simulink library "Plane_Movement_walk_right"  (R2024a)
settings: Solver=VariableStepAuto  StartTime=0.0  StopTime=10.0  RelTol=1e-3
undefined symbols (not defined in the file): Lower_limbs, Upper_limbs
libraries: functionAnglesSide x2, functionBezier_forward x1
settings Model: Creator=renre  LastModifiedBy=renre

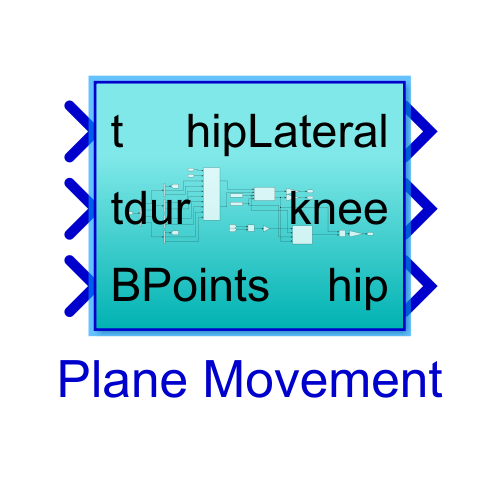
[thumbnail: Simulink's stored preview of the top-level diagram]
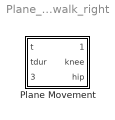
== system Plane_Movement_walk_right ==
  Plane Movement : Subsystem

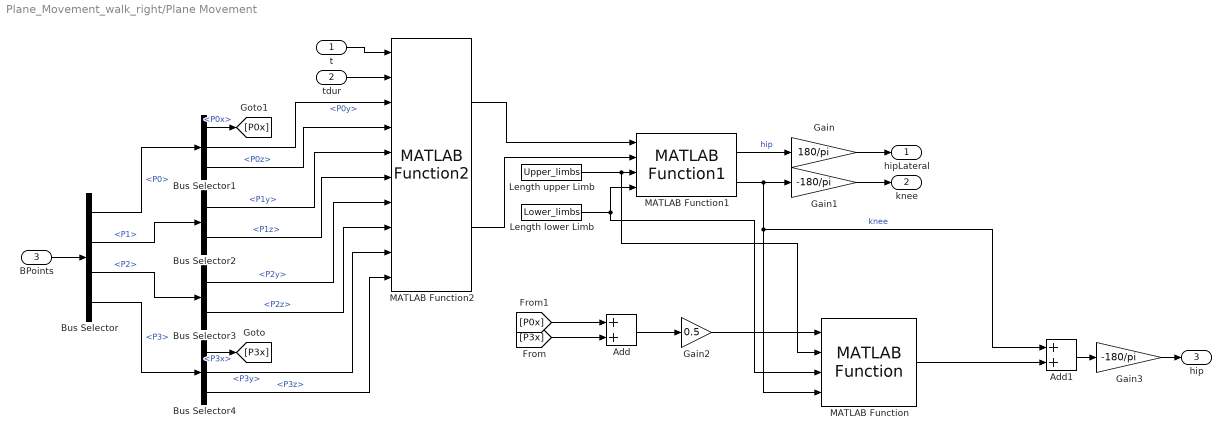
== system Plane_Movement_walk_right/Plane Movement ==
  t : Inport
  tdur : Inport  Port=2
  BPoints : Inport  Port=3
  Add : Sum
  Add1 : Sum
  Bus Selector : BusSelector  OutputSignals=P0,P1,P2,P3
  Bus Selector1 : BusSelector  OutputSignals=P0x,P0y,P0z
  Bus Selector2 : BusSelector  OutputSignals=P1y,P1z
  Bus Selector3 : BusSelector  OutputSignals=P2y,P2z
  Bus Selector4 : BusSelector  OutputSignals=P3x,P3y,P3z
  Gain : Gain  Gain=180/pi
  Gain1 : Gain  Gain=-180/pi
  Gain2 : Gain  Gain=0.5
  Gain3 : Gain  Gain=-180/pi
  Length lower Limb : Constant  Value=Lower_limbs
  Length upper Limb : Constant  Value=Upper_limbs
  MATLAB Function : functionAnglesSide/MATLAB Function  SystemSampleTime=-1  VariantActivationTime=update diagram  AllowFlexibleInterface=on  Latency=0  AutoFrameSizeCalculation=off
  MATLAB Function1 : functionAnglesSide/MATLAB Function1  SystemSampleTime=-1  VariantActivationTime=update diagram  AllowFlexibleInterface=on  Latency=0  AutoFrameSizeCalculation=off
  MATLAB Function2 : functionBezier_forward/MATLAB Function2  SystemSampleTime=-1  VariantActivationTime=update diagram  AllowFlexibleInterface=on  Latency=0  AutoFrameSizeCalculation=off
  hipLateral : Outport
  knee : Outport  Port=2
  hip : Outport  Port=3
  wires:
  Bus Selector2/2 -> MATLAB Function2/6  "<P1z>"
  Bus Selector/1 -> Bus Selector1/1  "<P0>"
  Bus Selector1/2 -> MATLAB Function2/3  "<P0y>"
  BPoints/1 -> Bus Selector/1
  Bus Selector/2 -> Bus Selector2/1  "<P1>"
  Bus Selector4/3 -> MATLAB Function2/10  "<P3z>"
  Bus Selector/4 -> Bus Selector4/1  "<P3>"
  Bus Selector1/3 -> MATLAB Function2/4  "<P0z>"
  Bus Selector4/2 -> MATLAB Function2/9  "<P3y>"
  Bus Selector3/1 -> MATLAB Function2/7  "<P2y>"
  Bus Selector2/1 -> MATLAB Function2/5  "<P1y>"
  Bus Selector3/2 -> MATLAB Function2/8  "<P2z>"
  Bus Selector/3 -> Bus Selector3/1  "<P2>"
  MATLAB Function2/2 -> MATLAB Function1/2
  MATLAB Function2/1 -> MATLAB Function1/1
  MATLAB Function1/2 -> Add1/1, MATLAB Function/4, Gain1/1  "knee"
  tdur/1 -> MATLAB Function2/2
  MATLAB Function1/1 -> Gain/1  "hip"
  t/1 -> MATLAB Function2/1
  Length upper Limb/1 -> MATLAB Function/2, MATLAB Function1/3
  Length lower Limb/1 -> MATLAB Function/3, MATLAB Function1/4
  Gain1/1 -> knee/1
  Gain/1 -> hipLateral/1
  Gain2/1 -> MATLAB Function/1
  Add/1 -> Gain2/1
  [P0x] -> Add/1
  [P3x] -> Add/2
  MATLAB Function/1 -> Add1/2
  Bus Selector4/1 -> [P3x]  "<P3x>"
  Bus Selector1/1 -> [P0x]  "<P0x>"
  Add1/1 -> Gain3/1
  Gain3/1 -> hip/1
